simulink model "AUAV_V3_TestSensors"  (R2015a)
settings: Solver=FixedStepDiscrete  StartTime=0.0  StopTime=10.0  FixedStep=T  RelTol=1e-3
PreLoadFcn:
  | %T = 0.0025;
  | MavlinkBus;
  | mcuInit;
  | % Baro Altitude Computation
  | % =========================
  | basePressure = 98192.64;
  | baseTemp = 288.215;
  | lapseRate = -0.00198122;
  | baseHeight = 0;
undefined symbols (not defined in the file): A0, A14, A15, A2, A3, A4, A5, A6, accBiasRateLimit, apSampleTime, B0, bankCommandLimit, barAdjust, baroCutoff, baroCutTemp, baroOffset, baroScale, barTGain1, barTGain2, barTMean1, barTMean2, bda, bde, bdr, bdt, bICda, bICde, bICdr, bICdt, cubeAccelGain16405, cubeGyroGain16405, cubeMagGain16405, D0, D11, D7, D8, daLimit, data, daTrimMax, daTrimMin, deLimit, derivativesConstant, deTrimMax, deTrimMin, drLimit, drTrimMax, drTrimMin, dtLimit, dtTrimMax, dtTrimMin, F2, F3, G0, G13, G15, gaind, GS_location, gyroBiasRateLimit, IC1max, imuOffset_xacc ... (+77)
libraries: MCHP_Blockset x158, simulink x84, SLUGS_Library x31, aerolibconvert2 x6, aerolibutil x4, aerolibtransform2 x3, dspmtrx3 x2, aerolibobsolete x2
(part 6 of 23)

== system AUAV_V3_TestSensors/Servo In Out ==
  Bias : Bias  Bias=-round(IC1max/2)
  Bias1 : Bias  Bias=-round(IC1max/2)
  Bias2 : Bias  Bias=+round(IC1max/2)
  Bias3 : Bias  Bias=+round(IC1max/2)
  Constant : Constant  Value=99
  Convert to Microseconds : Subsystem
  Convert to Microseconds1 : Subsystem
  Convert to Microseconds2 : Subsystem
  Data Type Conversion2 : DataTypeConversion  OutDataTypeStr=uint16  ConvertRealWorld=Stored Integer (SI)  RndMeth=Simplest
  Data Type Conversion3 : DataTypeConversion  OutDataTypeStr=uint16  ConvertRealWorld=Stored Integer (SI)  RndMeth=Simplest
  Data Type Conversion4 : DataTypeConversion  OutDataTypeStr=int16  ConvertRealWorld=Stored Integer (SI)  RndMeth=Simplest
  Data Type Conversion5 : DataTypeConversion  OutDataTypeStr=int16  ConvertRealWorld=Stored Integer (SI)  RndMeth=Simplest
  Input Capture RC Receiver1 : MCHP_Blockset/Pulse Input//Output/Input Capture  IntPriority=7  Channel="[1     2     3     4     5     6     7     8]"  Channel_OLD="[1  2  3  4  5  6  7  8]"  PIN_IC1=Dynamic Options  PIN_IC1_TXT=D0 / P64 / Pin[72]  PIN_IC2=Dynamic Options  PIN_IC2_TXT=D8 / P72 / Pin[68]  PIN_IC3=Dynamic Options  PIN_IC3_TXT=D11 / P75 / Pin[71]  PIN_IC4=Dynamic Options  PIN_IC4_TXT=A15 / P31 / Pin[67]  PIN_IC5=Dynamic Options  PIN_IC5_TXT=A5 / P21 / Pin[61]  PIN_IC6=Dynamic Options  PIN_IC6_TXT=A14 / P30 / Pin[66]  PIN_IC7=Dynamic Options  PIN_IC7_TXT=A0 / P16 / Pin[17]  PIN_IC8=Dynamic Options  PIN_IC8_TXT=A0 / P16 / Pin[17]  PIN_IC9=Dynamic Options  PIN_IC9_TXT=A0 / P16 / Pin[17]  PIN_IC10=Dynamic Options  PIN_IC10_TXT=A0 / P16 / Pin[17]  PIN_IC11=Dynamic Options  PIN_IC11_TXT=A0 / P16 / Pin[17]  PIN_IC12=Dynamic Options  PIN_IC12_TXT=A0 / P16 / Pin[17]  PIN_IC13=Dynamic Options  PIN_IC13_TXT=A0 / P16 / Pin[17]  PIN_IC14=Dynamic Options  PIN_IC14_TXT=A0 / P16 / Pin[17]  PIN_IC15=Dynamic Options  PIN_IC15_TXT=A0 / P16 / Pin[17]  PIN_IC16=Dynamic Options  PIN_IC16_TXT=A0 / P16 / Pin[17]  Channel_UP_Down_Periode="[1     1     1     1     1     1     1     1]"  MaxChannel="[0.003   0.003   0.003   0.003   0.003   0.003   0.003   0.003]"  SafeMarge="[0     0     0     0     0     0     0     0]"  MaxChannelValue="2.^[ 14.680  14.680  14.680  14.680  14.680  14.680  14.680  14.680]  =>  [26249  26249  26249  26249  26249  26249  26249  26249]"  ICxmax="[26249  26249  26249  26249  26249  26249  26249  26249]"  Timer="[1  1  1  1  1  1  1  1]"  ChangeDetected="[0     0     0     0     0     0     0     0]"  ChangeDetectedPortRef=3  SampleTime=.02  Status=OK  MCHP_PORT={Input Capture 1}{IC1}6:0:P64;{Input Capture 2}{IC2}6:0:P72;{Input Capture 3}{IC3}6:0:P75;{Input Capture 4}{IC4}6:0:P31;{Input Capture 5}{IC5}6:0:P21;{Input Capture 6}{IC6}6:0:P30;{Input Capture 7}{IC7}6:0:P16;{Input Capture 8}{IC8}6:0:P16;  MCHP_TIMER_REQUEST="{Input Capture 1}{IC1}6:0:1:0:[1  2  3  4  5]:210000;{Input Capture 1}{IC1}6:0:1:0:[1  2  3  4  5]:210000;{Input Capture 1}{IC1}6:0:1:0:[1  2  3  4  5]:210000;{Input Capture 1}{IC1}6:0:1:0:[1  2  3  4  5]:210000;{Input Capture 1}{IC1}6:0:1:0:[1  2  3  4  5]:210000;{Input Capture 1}{IC1}6:0:1:0:[1  2  3  4  5]:210000;{Input Capture 1}{IC1}6:0:1:0:[1  2  3  4  5]:210000;{Input Capture 1}{IC1}6:0:1:0:[1  2  3  4  5]:210000;"  MCHP_TIMER_RESULT=[1 26249.000000000011 ;1 26249.000000000011 ;1 26249.000000000011 ;1 26249.000000000011 ;1 26249.000000000011 ;1 26249.000000000011 ;1 26249.000000000011 ;1 26249.000000000011 ]  MCHP_MASTERLINK=|
      | AUAV_V3_TestSensors/Microchip Master
      | AUAV V3 Board
      | Busy Flag on D2 (RA6)
  Mixing : Subsystem
  Output Compare - HW Drive Servo motor : MCHP_Blockset/Pulse Input//Output/Output Compare - HW  Channel="[1     2]"  Channel_OLD="[1     2]"  PIN_OC1=Dynamic Options  PIN_OC1_TXT=G0 / P112 / Pin[90]  PIN_OC2=Dynamic Options  PIN_OC2_TXT=E0 / P80 / Pin[93]  PIN_OC3=Dynamic Options  PIN_OC3_TXT=D0 / P64 / Pin[72]  PIN_OC4=Dynamic Options  PIN_OC4_TXT=D0 / P64 / Pin[72]  PIN_OC5=Dynamic Options  PIN_OC5_TXT=D0 / P64 / Pin[72]  PIN_OC6=Dynamic Options  PIN_OC6_TXT=D0 / P64 / Pin[72]  PIN_OC7=Dynamic Options  PIN_OC7_TXT=D0 / P64 / Pin[72]  PIN_OC8=Dynamic Options  PIN_OC8_TXT=D0 / P64 / Pin[72]  PIN_OC9=Dynamic Options  PIN_OC9_TXT=D0 / P64 / Pin[72]  PIN_OC10=Dynamic Options  PIN_OC10_TXT=D0 / P64 / Pin[72]  PIN_OC11=Dynamic Options  PIN_OC11_TXT=D0 / P64 / Pin[72]  PIN_OC12=Dynamic Options  PIN_OC12_TXT=D0 / P64 / Pin[72]  PIN_OC13=Dynamic Options  PIN_OC13_TXT=D0 / P64 / Pin[72]  PIN_OC14=Dynamic Options  PIN_OC14_TXT=D0 / P64 / Pin[72]  PIN_OC15=Dynamic Options  PIN_OC15_TXT=D0 / P64 / Pin[72]  PIN_OC16=Dynamic Options  PIN_OC16_TXT=D0 / P64 / Pin[72]  PIN_OCFA=Dynamic Options  PIN_OCFA_TXT=A0 / P16 / Pin[17]  PIN_OCFB=Dynamic Options  PIN_OCFB_TXT=A0 / P16 / Pin[17]  PIN_OCFC=Dynamic Options  PIN_OCFC_TXT=A0 / P16 / Pin[17]  Channel_UP_Down_Periode="[5     5]"  PulseTrig=Single pulse triggered by block execution  InputPeriod=are set to the Max time (constant below)  MaxChannel="[0.003   0.003]"  MaxChannelUnique=.0001  MaxChannelValue="2.^[ 14.680  14.680]  =>  [26249  26249]"  OCxmax="[26249  26249]"  Timer="[1  1]"  SampleTime=.02  MCHP_PORT={Output Compare 1}{OC1}7:1:P112;{Output Compare 2}{OC2}7:1:P80;  MCHP_TIMER_REQUEST="{Output Compare 1}{OC1}7:0:1:0:[1  2  3  4  5]:210000;{Output Compare 1}{OC1}7:0:1:0:[1  2  3  4  5]:210000;"  MCHP_TIMER_RESULT=[1 26249.000000000011 ;1 26249.000000000011 ]  MCHP_MASTERLINK=|
      | AUAV_V3_TestSensors/Microchip Master
      | AUAV V3 Board
      | Busy Flag on D2 (RA6)
  Saturation : Saturate  UpperLimit=OC1max*2.2/3  LowerLimit=OC1max*0.8/3  RndMeth=Simplest
  Saturation1 : Saturate  UpperLimit=OC1max*2.2/3  LowerLimit=OC1max*0.8/3  RndMeth=Simplest
  mlNavigation : DataStoreWrite  DialogController=Simulink.DDGSource  DataStoreName=mlPwmCommands  DataStoreElements=mlPwmCommands.servo1_raw#mlPwmCommands.servo2_raw#mlPwmCommands.servo3_raw#mlPwmCommands.servo4_raw#mlPwmCommands.servo5_raw#mlPwmCommands.servo6_raw#mlPwmCommands.servo7_raw#mlPwmCommands.servo8_raw
  Out1 : Outport
  Out2 : Outport  Port=2
  Out3 : Outport  Port=3
  Out4 : Outport  Port=4
  Out5 : Outport  Port=5
  Out6 : Outport  Port=6
  wires:
  Input Capture RC Receiver1/1 -> Data Type Conversion4/1  "cmd PITCH raw"
  Input Capture RC Receiver1/4 -> Data Type Conversion5/1  "cmd ROLL raw"
  Bias/1 -> Mixing/1(Pitch)
  Bias1/1 -> Mixing/2(Roll)
  Bias2/1 -> Data Type Conversion2/1
  Bias3/1 -> Data Type Conversion3/1
  Saturation1/1 -> Convert to Microseconds1/1(PWM), Output Compare - HW Drive Servo motor/2
  Saturation/1 -> Convert to Microseconds/1(PWM), Output Compare - HW Drive Servo motor/1
  Mixing/2(Cmd Servo Right) -> Bias3/1
  Mixing/1(Cmd Servo Left) -> Bias2/1
  Data Type Conversion4/1 -> Bias/1
  Data Type Conversion5/1 -> Bias1/1
  Data Type Conversion3/1 -> Saturation1/1
  Data Type Conversion2/1 -> Saturation/1
  Input Capture RC Receiver1/2 -> Out1/1
  Input Capture RC Receiver1/3 -> Out2/1
  Input Capture RC Receiver1/5 -> Out3/1
  Input Capture RC Receiver1/6 -> Out4/1
  Input Capture RC Receiver1/7 -> Out5/1
  Input Capture RC Receiver1/8 -> Out6/1
  Constant/1 -> Convert to Microseconds2/1(PWM)
  Convert to Microseconds/1(uS) -> mlNavigation/1
  Convert to Microseconds1/1(uS) -> mlNavigation/2
  Convert to Microseconds2/1(uS) -> mlNavigation/5, mlNavigation/4, mlNavigation/3, mlNavigation/8, mlNavigation/7, mlNavigation/6
